simulink model "hybrid_cont"  (Simulink 6.0)
settings: Solver=ode45  StartTime=0.0  StopTime=10  RelTol=1e-3
libraries: simulink x3
settings Model: LastModifiedBy=c

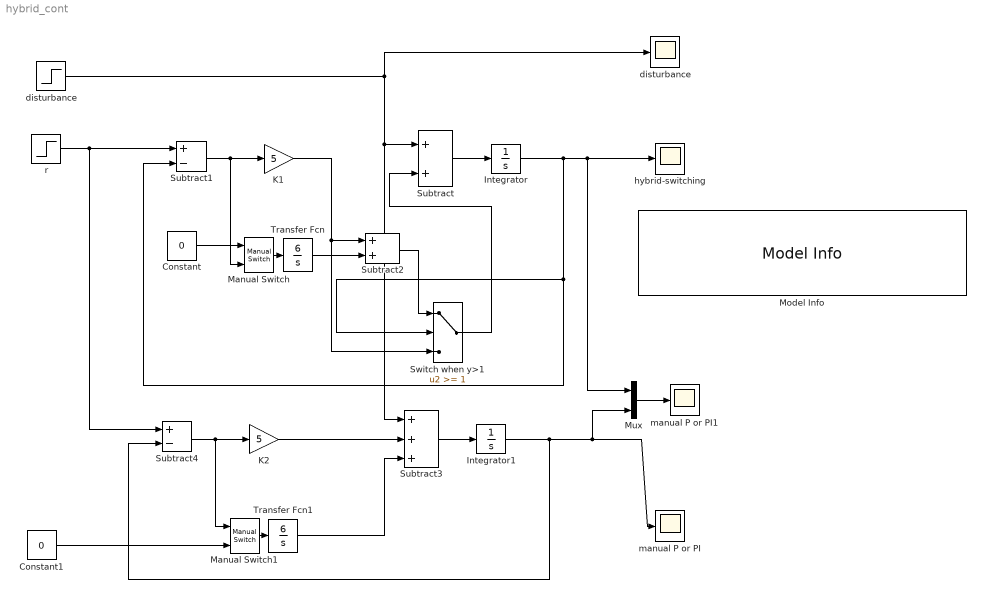
== system hybrid_cont ==
  Constant : Constant  Value=0
  Constant1 : Constant  Value=0
  Integrator : Integrator
  Integrator1 : Integrator
  K1 : Gain  Gain=5
  K2 : Gain  Gain=5
  Manual Switch : simulink/Signal Routing/Manual Switch  sw=0  action=0
  Manual Switch1 : simulink/Signal Routing/Manual Switch  sw=1  action=0
  Model Info : simulink/Model-Wide Utilities/Model Info  InitialBlockCM=None  BlockCM=None  Frame=on  DisplayStringWithTags=|  HorizontalTextAlignment=Left  LeftAlignmentValue=0.02  SourceBlockDiagram=hybrid_cont  TagMaxNumber=20
      | A. Feuer, G.C. Goodwin, M. Salgado, 
      | Potentia benefits of hybrid control for linear time invariant plants 
      | Proceedings of ACC, 
      | June 1997,p 2790-2794.\n
      | %<LastModificationDate>
  Mux : Mux  Inputs=2
  Subtract : Sum  OutScaling=2^-10
  Subtract1 : Sum  Inputs=+-  OutScaling=2^-10
  Subtract2 : Sum  OutScaling=2^-10
  Subtract3 : Sum  Inputs=+++  OutScaling=2^-10
  Subtract4 : Sum  Inputs=+-  OutScaling=2^-10
  Switch when y>1 : Switch  Threshold=1
  Transfer Fcn : TransferFcn  Numerator=[6]  Denominator=[1 0]
  Transfer Fcn1 : TransferFcn  Numerator=[6]  Denominator=[1 0]
  disturbance : Step  Time=5  After=-1  SampleTime=0
  "disturbance  " : Scope
  hybrid-switching : Scope
      settings: YMin=0.95  YMax=1.05
  manual P or PI : Scope
      settings: YMin=0.95  YMax=1.05  SaveName=ScopeData3
  manual P or PI1 : Scope
      settings: YMin=0.95  YMax=1.05  SaveName=ScopeData2
  r : Step  Time=0  SampleTime=0
  wires:
  Subtract1/1 -> K1/1, Manual Switch/1
  Subtract/1 -> Integrator/1
  Integrator/1 -> Subtract1/2, Switch when y>1/2, hybrid-switching/1, Mux/1
  Constant/1 -> Manual Switch/2
  Manual Switch/1 -> Transfer Fcn/1
  disturbance/1 -> "disturbance  "/1, Subtract/1, Subtract3/1
  r/1 -> Subtract1/1, Subtract4/1
  Switch when y>1/1 -> Subtract/2
  K1/1 -> Subtract2/1, Switch when y>1/3
  Transfer Fcn/1 -> Subtract2/2
  Subtract2/1 -> Switch when y>1/1
  Subtract4/1 -> K2/1, Manual Switch1/1
  Subtract3/1 -> Integrator1/1
  Integrator1/1 -> Subtract4/2, manual P or PI/1, Mux/2
  Constant1/1 -> Manual Switch1/2
  Manual Switch1/1 -> Transfer Fcn1/1
  Transfer Fcn1/1 -> Subtract3/3
  K2/1 -> Subtract3/2
  Mux/1 -> manual P or PI1/1
